simulink model "Simulation1"  (R2024a)
settings: Solver=VariableStepAuto  StartTime=0.0  StopTime=10.0  RelTol=1e-3
settings Model: Creator=Jeffery  LastModifiedBy=Jeffery

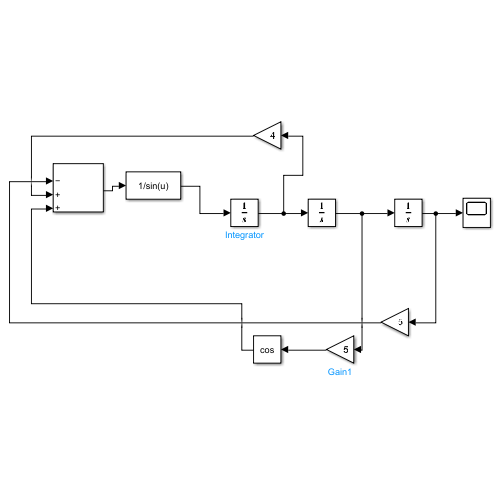
[thumbnail: Simulink's stored preview of the top-level diagram]
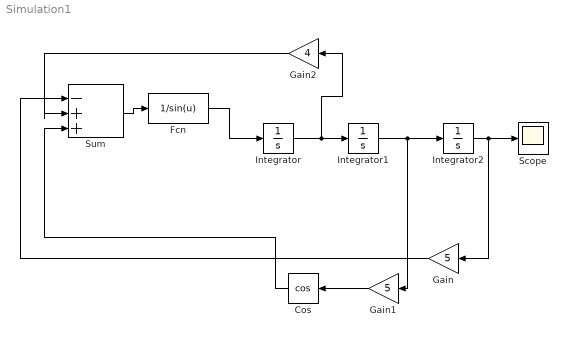
== system Simulation1 ==
  Cos : Trigonometry  Operator=cos
  Fcn : Fcn  Expr=1/sin(u)
  Gain : Gain  Gain=5
  Gain1 : Gain  Gain=5
  Gain2 : Gain  Gain=4
  Integrator : Integrator
  Integrator1 : Integrator
  Integrator2 : Integrator
  Scope : Scope
  Sum : Sum  Inputs=|-++
  wires:
  Integrator/1 -> Gain2/1, Integrator1/1
  Integrator1/1 -> Gain1/1, Integrator2/1
  Integrator2/1 -> Gain/1, Scope/1
  Sum/1 -> Fcn/1
  Fcn/1 -> Integrator/1
  Gain1/1 -> Cos/1
  Cos/1 -> Sum/3
  Gain2/1 -> Sum/2
  Gain/1 -> Sum/1
